simulink model "simulation_model_dynamic"  (R2024b)
settings: Solver=VariableStepAuto  StartTime=0.0  StopTime=100  MaxStep=1/60  RelTol=1e-3  EnableMultiTasking=on
values from neighbouring files (symbols this model uses):
  c_f = c_f*Cb    [fun00_GFL_pu_2_normial.m]    (also in fun00_GFM_pu_2_normial.m)
  fb = 60    [case_data.m]    (also in sim_m_case1.m; sim_m_case1_bench.m; sim_m_case2.m; sim_m_case2_bench.m)
  ki_i = ki_i_pu*Vb_p_ph/Ib_p_ph    [fun00_GFL_pu_2_normial.m]    (also in fun00_GFM_pu_2_normial.m)
  ki_p = ki_p_pu/Sb*Ib_p_ph    [fun00_GFL_pu_2_normial.m]
  ki_pll = ki_pll/Vb_p_ph    [fun00_GFL_pu_2_normial.m]
  ki_q = ki_q_pu/Sb*Ib_p_ph    [fun00_GFL_pu_2_normial.m]
  kp_i = kp_i_pu*Vb_p_ph/Ib_p_ph    [fun00_GFL_pu_2_normial.m]    (also in fun00_GFM_pu_2_normial.m)
  kp_p = kp_p_pu/Sb*Ib_p_ph    [fun00_GFL_pu_2_normial.m]
  kp_pll = kp_pll/Vb_p_ph    [fun00_GFL_pu_2_normial.m]
  kp_q = kp_q_pu/Sb*Ib_p_ph    [fun00_GFL_pu_2_normial.m]
  l_f = l_f*Lb    [fun00_GFL_pu_2_normial.m]    (also in fun00_GFM_pu_2_normial.m)
  line = mpc.line    [sim_m_case1.m]    (also in sim_m_case1_bench.m; sim_m_case2.m = mpc.line*1.1; sim_m_case2_bench.m = mpc.line*1.1; sim_m_case2_sparse.m = mpc.line*1.1)
  pset = p_set_pu*Sb    [fun00_GFL_pu_2_normial.m]
  qset = q_set_pu*Sb    [fun00_GFL_pu_2_normial.m]
  r_f = r_f*Zb    [fun00_GFL_pu_2_normial.m]    (also in fun00_GFM_pu_2_normial.m)
  Sb = 100*10^6    (= 100000000)    [sim_m_case1.m]    (also in sim_m_case1_bench.m; sim_m_case2.m; sim_m_case2_bench.m; sim_m_case2_sparse.m)
  t_gfl = 35    [sim_m_case1.m]    (also in sim_m_case1_bench.m = 30; sim_m_case2.m; sim_m_case2_bench.m = 30; sim_m_case2_sparse.m)
  t_gfm = 30    [sim_m_case1.m]    (also in sim_m_case1_bench.m; sim_m_case2.m; sim_m_case2_bench.m; sim_m_case2_sparse.m)
  trans_l = mpc.trans_l    [sim_m_case1.m]    (also in sim_m_case1_bench.m; sim_m_case2.m; sim_m_case2_bench.m; sim_m_case2_sparse.m)
  Vb_gfm = 20*10^3    (= 20000)    [sim_m_case1.m]    (also in sim_m_case1_bench.m; sim_m_case2.m; sim_m_case2_bench.m; sim_m_case2_sparse.m)
  Vb_h = 230*10^3    (= 230000)    [sim_m_case1.m]    (also in sim_m_case1_bench.m; sim_m_case2.m; sim_m_case2_bench.m; sim_m_case2_sparse.m)
  Vdc = 3*Vb_p_ph    [fun00_GFL_pu_2_normial.m]    (also in fun00_GFM_pu_2_normial.m)
  wb = 2*pi*fb    (= 376.991118431)    [case_data.m]    (also in sim_m_case1.m; sim_m_case1_bench.m; sim_m_case2.m; sim_m_case2_bench.m)
undefined symbols (not defined in the file or in its folder): c_f_gfm, d_gfl, D_p_gfm, D_p_gfm_s, D_q_gfm, DiscIntNeverNeededParam, Init, Init_GFL, J_gfm, ki_i_gfm, ki_pll_s, ki_vc_gfm, kp_i_gfm, kp_pll_s, kp_vc_gfm, l_f_gfm, P_set_gfm, Q_set_gfm, r_f_gfm, Vb, Vdc_gfm, VSM
libraries: spsThreePhaseVIMeasurementLib x52, spsabctodq0Lib x48, slpidlib x42, spsThreePhaseSeriesRLCBranchLib x36, spsFirstOrderFilterLib x16, spsThreePhaseTransformerTwoWindingsLib x9, spsGroundLib x9, spsPowerPositiveSequenceLib x9, spsdq0toabcLib x9, spsUniversalBridgeLib x9, spsDCVoltageSourceLib x9, spsThreePhaseSourceLib x5
(part 1 of 8)
settings Model: SimulationMode=accelerator  Creator=MathWorks  LastModifiedBy=victo
settings SolverCC: AlgebraicLoopSolver=TrustRegion
settings DataIOCC: SaveFormat=Array  SignalLoggingSaveFormat=ModelDataLogs  SaveOutput=off  SaveTime=off  ReturnWorkspaceOutputs=off  TimeSaveName=t  SignalLoggingName=sigsOut
settings OptimizationCC: BlockReduction=off  BooleanDataType=off  ExpressionDepthLimit=2147483647  InitFltsAndDblsToZero=on  LifeSpan=inf
settings DebuggingCC: UnderspecifiedInitializationDetection=Classic  MergeDetectMultiDrivingBlocksExec=none  SignalResolutionControl=TryResolveAllWithWarning  MultiTaskDSMMsg=warning  MultiTaskCondExecSysMsg=none  FcnCallInpInsideContextMsg=warning  StateNameClashWarn=warning  SFUnexpectedBacktrackingDiag=warning  SFNoUnconditionalDefaultTransitionDiag=warning  SFExecutionAtInitializationDiag=none  ArithmeticOperatorsInVariantConditions=warning
settings HardwareCC: ProdBitPerPointer=32  ProdBitPerSizeT=32  ProdBitPerPtrDiffT=32  ProdLargestAtomicFloat=None  ProdIntDivRoundTo=Undefined  ProdEndianess=Unspecified  ProdWordSize=32  ProdHWDeviceType=32-bit Generic  TargetBitPerPointer=64  TargetBitPerSizeT=64  TargetBitPerPtrDiffT=64  TargetLongLongMode=on  TargetIntDivRoundTo=Zero  TargetEndianess=LittleEndian  TargetWordSize=64  TargetHWDeviceType=MATLAB Host  ProdEqTarget=off
settings ModelReferenceCC: EnableRefExpFcnMdlSchedulingChecks=on  PropagateSignalLabelsOutOfModel=off
settings SFSimCC: SimUseLocalCustomCode=off  CustomCodeUndefinedFunction=UseInterfaceOnly
settings RTWCC: RTWUseLocalCustomCode=off  GPUComputeCapability=3.5
settings CodeAppCC: StateflowObjectComments=on
settings GRTTargetCC: TargetLangStandard=C89/C90 (ANSI)  CombineOutputUpdateFcns=off  GRTInterface=on
settings ConfigComp: CovMetricSettings=dw  CovSaveCumulativeToWorkspaceVar=on  CovSaveSingleToWorkspaceVar=on  CovExternalEMLEnable=off  CovSFcnEnable=off
settings SimscapeCC: SimscapeNormalizeSystem=off

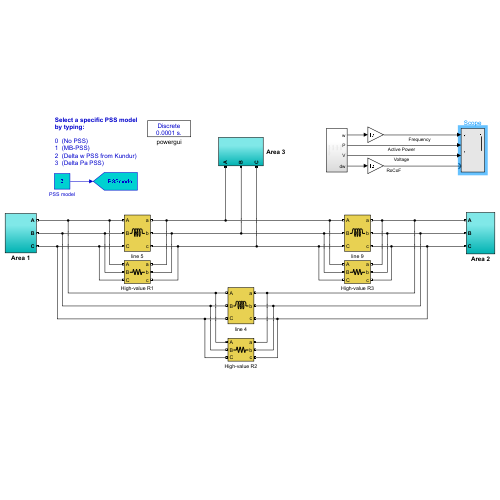
[thumbnail: Simulink's stored preview of the top-level diagram]
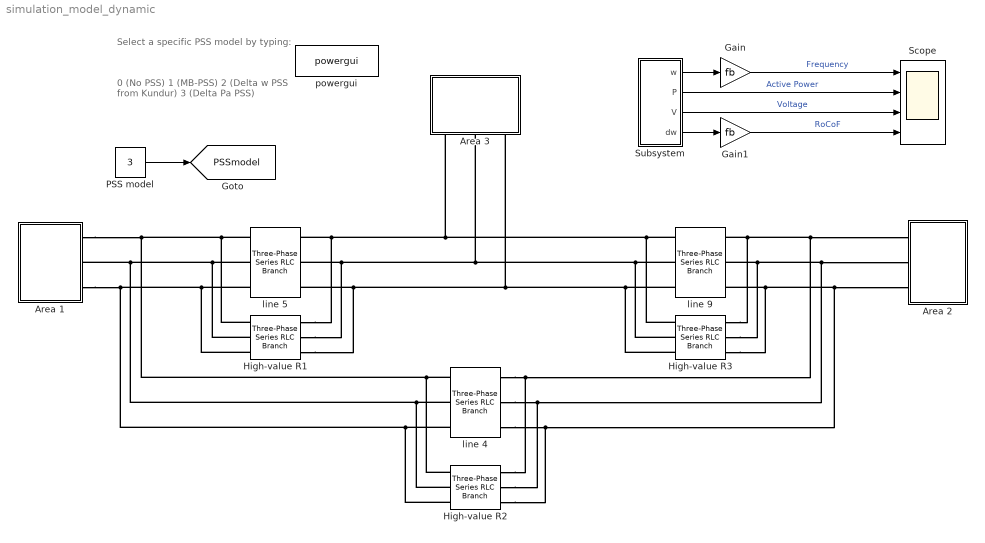
== system simulation_model_dynamic ==
  note: Select a specific PSS model
      | by typing:
  note: 0  (No PSS)
      | 1  (MB-PSS)
      | 2  (Delta w PSS from Kundur)
      | 3  (Delta Pa PSS)
  Area 1 : Subsystem
  Area 2 : Subsystem
  Area 3 : Subsystem
  Gain : Gain  Gain=fb
  Gain1 : Gain  Gain=fb
  High-value R1 : spsThreePhaseSeriesRLCBranchLib/Three-Phase Series RLC Branch  LConnTagsString=A|B|C  RConnTagsString=A|B|C  BranchType=R  Resistance=1e6  Inductance=line(3,4)  Capacitance=1e-6  Measurements=None
  High-value R2 : spsThreePhaseSeriesRLCBranchLib/Three-Phase Series RLC Branch  LConnTagsString=A|B|C  RConnTagsString=A|B|C  BranchType=R  Resistance=1e6  Inductance=line(3,4)  Capacitance=1e-6  Measurements=None
  High-value R3 : spsThreePhaseSeriesRLCBranchLib/Three-Phase Series RLC Branch  LConnTagsString=A|B|C  RConnTagsString=A|B|C  BranchType=R  Resistance=1e6  Inductance=line(3,4)  Capacitance=1e-6  Measurements=None
  PSS model : Constant  Value=3
  Scope : Scope  NumInputPorts=4
  Subsystem : Subsystem
  line 4 : spsThreePhaseSeriesRLCBranchLib/Three-Phase Series RLC Branch  LConnTagsString=A|B|C  RConnTagsString=A|B|C  BranchType=L  Resistance=line(14,3)  Inductance=line(4,4)  Capacitance=1e-6  Measurements=None
  line 5 : spsThreePhaseSeriesRLCBranchLib/Three-Phase Series RLC Branch  LConnTagsString=A|B|C  RConnTagsString=A|B|C  BranchType=L  Resistance=1e-4  Inductance=line(5,4)  Capacitance=1e-6  Measurements=None
  line 9 : spsThreePhaseSeriesRLCBranchLib/Three-Phase Series RLC Branch  LConnTagsString=A|B|C  RConnTagsString=A|B|C  BranchType=L  Resistance=line(14,3)  Inductance=line(9,4)  Capacitance=1e-6  Measurements=None
  powergui : sps_lib/powergui  Priority=2  SimulationMode=Discrete  SampleTime=1e-4  frequency=60  Iterations=1000  frequencyindice=0  Pbase=100e6  ErrMax=0.001  UnitsV=kV  UnitsW=MW  buscounter=0  FunctionMessages=off  echomessages=off  EnableUseOfTLC=off  CurrentSourceSwitches=off  DisableSnubberDevices=off  DisableRonSwitches=off  DisableVfSwitches=off  DisplayEquations=off  AutomaticDiscreteSolvers=off  SolverType=Tustin  Interpol=off  ExternalGateDelay=off  methode=off  Ts=0  x0status=steady  SPID=off  SwTol=0  HookPort=off  NonlinearTolerance=1e-4  nMaxIteration=100  ContinueOnMaxIteration=off  RestoreLinks=warning  ResistiveCurrentMeasurement=off  Frange=logspace(0,3,50)  Ylog=off  Xlog=off  ShowGrid=off  save=off  variable=ZData  structure=0  ZoomFFT=on  StartTime=0.0  cycles=1  DisplayStyle=1  fundamental=60  FreqAxis=off  MaxFrequency=1000  frequencyindicesteady=1  RmsSteady=2  display=off
  tag scope: PSSmodel=global
  wires:
  PSS model/1 -> [PSSmodel]
  Subsystem/2(P) -> Scope/2  "Active Power"
  Gain/1 -> Scope/1  "Frequency"
  Subsystem/3(V) -> Scope/3  "Voltage"
  Subsystem/1(w) -> Gain/1
  Subsystem/4(dw) -> Gain1/1
  Gain1/1 -> Scope/4  "RoCoF"
  connections:
  line 5/LConn2 -- High-value R1/LConn2 -- High-value R2/LConn2 -- line 4/LConn2 -- Area 1/RConn2
  line 5/LConn1 -- High-value R1/LConn1 -- High-value R2/LConn1 -- line 4/LConn1 -- Area 1/RConn1
  line 5/LConn3 -- High-value R1/LConn3 -- High-value R2/LConn3 -- line 4/LConn3 -- Area 1/RConn3
  line 4/RConn2 -- High-value R2/RConn2 -- Area 2/LConn2 -- High-value R3/RConn2 -- line 9/RConn2
  line 4/RConn1 -- High-value R2/RConn1 -- Area 2/LConn1 -- High-value R3/RConn1 -- line 9/RConn1
  line 4/RConn3 -- High-value R2/RConn3 -- Area 2/LConn3 -- High-value R3/RConn3 -- line 9/RConn3
  line 9/LConn2 -- High-value R3/LConn2 -- Area 3/LConn2 -- High-value R1/RConn2 -- line 5/RConn2
  line 9/LConn1 -- High-value R3/LConn1 -- Area 3/LConn1 -- High-value R1/RConn1 -- line 5/RConn1
  line 9/LConn3 -- High-value R3/LConn3 -- Area 3/LConn3 -- High-value R1/RConn3 -- line 5/RConn3

== system simulation_model_dynamic/Area 1 ==
  note: Area 1
  1 : spsThreePhaseVIMeasurementLib/Three-Phase V-I Measurement  VoltageMeasurement=phase-to-ground  SetLabelV=on  LabelV=Vabc_1  Vpu=off  VpuLL=off  CurrentMeasurement=no  SetLabelI=off  LabelI=Iabc  Ipu=off  Pbase=100e6  Vbase=500e3  OutputType=Complex  PhasorSimulation=off  PSBequivalent=0
  100MVA 20 kV-230 kV1 : spsThreePhaseTransformerTwoWindingsLib/Three-Phase Transformer (Two Windings)  Winding1Connection=Yg  Winding2Connection=Yg  CoreType=Three single-phase transformers  SetSaturation=off  Hysteresis=off  DataFile='hysteresis'  SetInitialFlux=off  Measurements=None  UNITS=pu  NominalPower="[ Sb   fb ]"  Winding1="[ 20e3  1e-6   0  ]"  Winding2="[ 230e3  1e-6   trans_l ]"  Rm=500  Lm=500  L0=0.5  Saturation="[ 0,0  ;  0.005,1.2  ;  1.0,1.4 ]"  InitialFluxes=[ 0.8 , -0.8 , 0.7 ]  BreakLoop=off  DiscreteSolver=Trapezoidal iterative  DataType=off  TransfoNumber=0
  100MVA 20 kV-230 kV2 : spsThreePhaseTransformerTwoWindingsLib/Three-Phase Transformer (Two Windings)  Winding1Connection=Yg  Winding2Connection=Yg  CoreType=Three single-phase transformers  SetSaturation=off  Hysteresis=off  DataFile='hysteresis'  SetInitialFlux=off  Measurements=None  UNITS=pu  NominalPower="[ Sb   fb ]"  Winding1="[ 20e3  1e-6   0  ]"  Winding2="[ 230e3  1e-6   trans_l ]"  Rm=500  Lm=500  L0=0.5  Saturation="[ 0,0  ;  0.005,1.2  ;  1.0,1.4 ]"  InitialFluxes=[ 0.8 , -0.8 , 0.7 ]  BreakLoop=off  DiscreteSolver=Trapezoidal iterative  DataType=off  TransfoNumber=0
  100MVA 20 kV-230 kV3 : spsThreePhaseTransformerTwoWindingsLib/Three-Phase Transformer (Two Windings)  Winding1Connection=Yg  Winding2Connection=Yg  CoreType=Three single-phase transformers  SetSaturation=off  Hysteresis=off  DataFile='hysteresis'  SetInitialFlux=off  Measurements=None  UNITS=pu  NominalPower="[Sb   fb ]"  Winding1="[ 20e3  1e-6   0  ]"  Winding2="[ 230e3  1e-6   trans_l ]"  Rm=500  Lm=500  L0=0.5  Saturation="[ 0,0  ;  0.005,1.2  ;  1.0,1.4 ]"  InitialFluxes=[ 0.8 , -0.8 , 0.7 ]  BreakLoop=off  DiscreteSolver=Trapezoidal iterative  DataType=off  TransfoNumber=0
  13 : spsThreePhaseVIMeasurementLib/Three-Phase V-I Measurement  VoltageMeasurement=phase-to-ground  SetLabelV=on  LabelV=Vabc_13  Vpu=off  VpuLL=off  CurrentMeasurement=no  SetLabelI=off  LabelI=Iabc  Ipu=off  Pbase=100e6  Vbase=500e3  OutputType=Complex  PhasorSimulation=off  PSBequivalent=0
  14 : spsThreePhaseVIMeasurementLib/Three-Phase V-I Measurement  VoltageMeasurement=phase-to-ground  SetLabelV=on  LabelV=Vabc_14  Vpu=off  VpuLL=off  CurrentMeasurement=no  SetLabelI=off  LabelI=Iabc  Ipu=off  Pbase=100e6  Vbase=500e3  OutputType=Complex  PhasorSimulation=off  PSBequivalent=0
  2 : spsThreePhaseVIMeasurementLib/Three-Phase V-I Measurement  VoltageMeasurement=phase-to-ground  SetLabelV=on  LabelV=Vabc_2  Vpu=off  VpuLL=off  CurrentMeasurement=no  SetLabelI=off  LabelI=Iabc  Ipu=off  Pbase=100e6  Vbase=500e3  OutputType=Complex  PhasorSimulation=off  PSBequivalent=0
  3 : spsThreePhaseVIMeasurementLib/Three-Phase V-I Measurement  VoltageMeasurement=phase-to-ground  SetLabelV=on  LabelV=Vabc_3  Vpu=off  VpuLL=off  CurrentMeasurement=no  SetLabelI=off  LabelI=Iabc  Ipu=off  Pbase=100e6  Vbase=500e3  OutputType=Complex  PhasorSimulation=off  PSBequivalent=0
  4 : spsThreePhaseVIMeasurementLib/Three-Phase V-I Measurement  VoltageMeasurement=phase-to-ground  SetLabelV=on  LabelV=Vabc_4  Vpu=off  VpuLL=off  CurrentMeasurement=no  SetLabelI=off  LabelI=Iabc  Ipu=off  Pbase=100e6  Vbase=500e3  OutputType=Complex  PhasorSimulation=off  PSBequivalent=0
  Bus Selector : BusSelector  OutputSignals="Mechanical.Rotor speed  wm  (pu),Output active power   Peo (pu),Output reactive power  Qeo (pu)"
  High-value R : spsThreePhaseSeriesRLCBranchLib/Three-Phase Series RLC Branch  LConnTagsString=A|B|C  RConnTagsString=A|B|C  BranchType=R  Resistance=1e6  Inductance=line(3,4)  Capacitance=1e-6  Measurements=None
  High-value R1 : spsThreePhaseSeriesRLCBranchLib/Three-Phase Series RLC Branch  LConnTagsString=A|B|C  RConnTagsString=A|B|C  BranchType=R  Resistance=1e6  Inductance=line(3,4)  Capacitance=1e-6  Measurements=None
  INVERTER 1 : Subsystem
  INVERTER 2 : Subsystem
  INVERTER 3 : Subsystem
  M1 100 MVA : spsSynchronousMachinepuStandardLib/Synchronous Machine pu Standard  PresetModel=No  MechanicalLoad=Mechanical power Pm  ShowDetailedParameters=on  RotorType=Round  Units=per unit standard parameters  MeasurementBus=off  NominalParameters="[100e6  20000   60 ]"  Reactances1=[1.8 .3 .25 1.7 .55 .25 .2]  Reactances2=[ 1.305, 0.296, 0.252, 0.474, 0.243, 0.18 ]  dAxisTimeConstants=Open-circuit  qAxisTimeConstants=Open-circuit  TimeConstants1=[]  TimeConstants2=[8 .03 .4 .05]  TimeConstants3=[]  TimeConstants4=[]  TimeConstants5=[ 1.01, 0.053, 0.1 ]  TimeConstants6=[]  TimeConstants7=[]  TimeConstants8=[]  StatorResistance=0.025  Mechanical=[1 0 4]  PolePairs=4  InitialConditions=[0 0 0 0 0 0 0 0 1.43051]  SetSaturation=off  Saturation=[0.6404,0.7127,0.8441,0.9214,0.9956,1.082,1.19,1.316,1.457;0.7,0.7698,0.8872,0.9466,0.9969,1.046,1.1,1.151,1.201]  LoadFlowParameters=[1 700000000 0 0 0]  TsPowergui=0  TsBlock=-1  IterativeModel=Trapezoidal non iterative  IterativeDiscreteModel=Trapezoidal non iterative  BusType=PV  Pref=50e6  Qref=0  Qmin=-Inf  Qmax=Inf  PLF=0  QLF=0
  M1: Turbine & Regulators : Subsystem
  Pref1 : Constant  Value=0.5
  Terminator : Terminator
  Terminator1 : Terminator
  Three-Phase Dynamic Load : spsThreePhaseDynamicLoadLib/Three-Phase Dynamic Load  NominalVoltage=[ Vb_h fb ]  ActiveReactivePowers=[400e6 0]  PositiveSequence=[1 0]  ExternalControl=off  NpNq=[0.7473 0.7268]  TimeConstants="[0  0.011  0  0.0366]"  MinimumVoltage=0.5  Tfilter=1e-4  LoadFlowParameters=[4,0,0,0,0]
      settings: LibrarySourceBlock=|
      | sps_lib/Passives/Three-Phase
      | Dynamic Load
  Three-Phase Dynamic Load1 : spsThreePhaseDynamicLoadLib/Three-Phase Dynamic Load  NominalVoltage=[ Vb_h fb ]  ActiveReactivePowers=[581e6 -100e6]  PositiveSequence=[0.994 -11.8]  ExternalControl=off  NpNq=[0.7473 0.7268]  TimeConstants="[0  0.011  0  0.0366]"  MinimumVoltage=0.5  Tfilter=1e-4  LoadFlowParameters=[4,0,0,0,0]
      settings: LibrarySourceBlock=|
      | sps_lib/Passives/Three-Phase
      | Dynamic Load
  Vref11 : Constant
  line 1 : spsThreePhaseSeriesRLCBranchLib/Three-Phase Series RLC Branch  LConnTagsString=A|B|C  RConnTagsString=A|B|C  BranchType=L  Resistance=1e-4  Inductance=line(1,4)  Capacitance=1e-6  Measurements=None
  line 3 : spsThreePhaseSeriesRLCBranchLib/Three-Phase Series RLC Branch  LConnTagsString=A|B|C  RConnTagsString=A|B|C  BranchType=L  Resistance=1e-4  Inductance=line(3,4)  Capacitance=1e-6  Measurements=None
  " A" : PMIOPort  Side=Right
  " B" : PMIOPort  Port=2  Side=Right
  " C" : PMIOPort  Port=3  Side=Right
  tag scope: P_sm1=global, Q_sm1=global, w_sm1=global
  wires:
  Pref1/1 -> M1: Turbine & Regulators/2(Pref)
  [PSSmodel] -> M1: Turbine & Regulators/4(PSS)
  M1: Turbine & Regulators/1(Pm) -> M1 100 MVA/1
  M1: Turbine & Regulators/2(Vf) -> M1 100 MVA/2
  Vref11/1 -> M1: Turbine & Regulators/3(Vref)
  M1 100 MVA/1 -> M1: Turbine & Regulators/1(m), Bus Selector/1
  Bus Selector/1 -> [w_sm1]  "<Rotor speed  wm  (pu)>"
  Bus Selector/2 -> [P_sm1]  "<Output active power   Peo (pu)>"
  Bus Selector/3 -> [Q_sm1]  "<Output reactive power  Qeo (pu)>"
  Three-Phase Dynamic Load/1 -> Terminator/1
  Three-Phase Dynamic Load1/1 -> Terminator1/1
  connections:
  2/LConn1 -- INVERTER 2/LConn1
  2/LConn3 -- INVERTER 2/LConn3
  100MVA 20 kV-230 kV3/RConn1 -- Three-Phase Dynamic Load1/LConn1 -- 4/LConn1 -- High-value R/RConn1 -- line 3/RConn1
  Three-Phase Dynamic Load1/LConn2 -- 4/LConn2 -- 100MVA 20 kV-230 kV3/RConn2 -- High-value R/RConn2 -- line 3/RConn2
  4/LConn3 -- Three-Phase Dynamic Load1/LConn3 -- 100MVA 20 kV-230 kV3/RConn3 -- High-value R/RConn3 -- line 3/RConn3
  INVERTER 1/LConn1 -- 13/LConn1
  INVERTER 1/LConn2 -- 13/LConn2
  INVERTER 1/LConn3 -- 13/LConn3
  line 3/LConn2 -- High-value R/LConn2 -- Three-Phase Dynamic Load/LConn2 -- 3/RConn2
  line 3/LConn1 -- High-value R/LConn1 -- Three-Phase Dynamic Load/LConn1 -- 3/RConn1
  3/LConn3 -- 100MVA 20 kV-230 kV2/RConn3 -- High-value R1/RConn3 -- line 1/RConn3
  2/LConn2 -- INVERTER 2/LConn2
  1/LConn1 -- 100MVA 20 kV-230 kV1/RConn1
  1/LConn2 -- 100MVA 20 kV-230 kV1/RConn2
  1/LConn3 -- 100MVA 20 kV-230 kV1/RConn3
  3/LConn1 -- 100MVA 20 kV-230 kV2/RConn1 -- High-value R1/RConn1 -- line 1/RConn1
  line 3/LConn3 -- High-value R/LConn3 -- Three-Phase Dynamic Load/LConn3 -- 3/RConn3
  3/LConn2 -- 100MVA 20 kV-230 kV2/RConn2 -- High-value R1/RConn2 -- line 1/RConn2
  100MVA 20 kV-230 kV1/LConn3 -- M1 100 MVA/RConn3 -- 13/RConn3
  100MVA 20 kV-230 kV1/LConn2 -- M1 100 MVA/RConn2 -- 13/RConn2
  100MVA 20 kV-230 kV1/LConn1 -- M1 100 MVA/RConn1 -- 13/RConn1
  100MVA 20 kV-230 kV2/LConn2 -- 2/RConn2
  100MVA 20 kV-230 kV2/LConn1 -- 2/RConn1
  100MVA 20 kV-230 kV2/LConn3 -- 2/RConn3
  4/RConn1 -- " A"/RConn1
  " B"/RConn1 -- 4/RConn2
  " C"/RConn1 -- 4/RConn3
  1/RConn1 -- High-value R1/LConn1 -- line 1/LConn1
  1/RConn2 -- High-value R1/LConn2 -- line 1/LConn2
  1/RConn3 -- High-value R1/LConn3 -- line 1/LConn3
  14/LConn1 -- INVERTER 3/LConn1
  14/LConn2 -- INVERTER 3/LConn2
  14/LConn3 -- INVERTER 3/LConn3
  14/RConn1 -- 100MVA 20 kV-230 kV3/LConn1
  100MVA 20 kV-230 kV3/LConn2 -- 14/RConn2
  14/RConn3 -- 100MVA 20 kV-230 kV3/LConn3

== system simulation_model_dynamic/Area 2 ==
  note: Area 2
  15 : spsThreePhaseVIMeasurementLib/Three-Phase V-I Measurement  VoltageMeasurement=phase-to-ground  SetLabelV=on  LabelV=Vabc_15  Vpu=off  VpuLL=off  CurrentMeasurement=no  SetLabelI=off  LabelI=Iabc  Ipu=off  Pbase=100e6  Vbase=500e3  OutputType=Complex  PhasorSimulation=off  PSBequivalent=0
  5 : spsThreePhaseVIMeasurementLib/Three-Phase V-I Measurement  VoltageMeasurement=phase-to-ground  SetLabelV=on  LabelV=Vabc_5  Vpu=off  VpuLL=off  CurrentMeasurement=no  SetLabelI=off  LabelI=Iabc  Ipu=off  Pbase=100e6  Vbase=500e3  OutputType=Complex  PhasorSimulation=off  PSBequivalent=0
  6 : spsThreePhaseVIMeasurementLib/Three-Phase V-I Measurement  VoltageMeasurement=phase-to-ground  SetLabelV=on  LabelV=Vabc_6  Vpu=off  VpuLL=off  CurrentMeasurement=no  SetLabelI=off  LabelI=Iabc  Ipu=off  Pbase=100e6  Vbase=500e3  OutputType=Complex  PhasorSimulation=off  PSBequivalent=0
  7 : spsThreePhaseVIMeasurementLib/Three-Phase V-I Measurement  VoltageMeasurement=phase-to-ground  SetLabelV=on  LabelV=Vabc_7  Vpu=off  VpuLL=off  CurrentMeasurement=no  SetLabelI=off  LabelI=Iabc  Ipu=off  Pbase=100e6  Vbase=500e3  OutputType=Complex  PhasorSimulation=off  PSBequivalent=0
  8 : spsThreePhaseVIMeasurementLib/Three-Phase V-I Measurement  VoltageMeasurement=phase-to-ground  SetLabelV=on  LabelV=Vabc_8  Vpu=off  VpuLL=off  CurrentMeasurement=no  SetLabelI=off  LabelI=Iabc  Ipu=off  Pbase=100e6  Vbase=500e3  OutputType=Complex  PhasorSimulation=off  PSBequivalent=0
  Bus Selector : BusSelector  OutputSignals="Mechanical.Rotor speed  wm  (pu),Output active power   Peo (pu),Output reactive power  Qeo (pu)"
  High-value R1 : spsThreePhaseSeriesRLCBranchLib/Three-Phase Series RLC Branch  LConnTagsString=A|B|C  RConnTagsString=A|B|C  BranchType=R  Resistance=1e6  Inductance=line(3,4)  Capacitance=1e-6  Measurements=None
  High-value R3 : spsThreePhaseSeriesRLCBranchLib/Three-Phase Series RLC Branch  LConnTagsString=A|B|C  RConnTagsString=A|B|C  BranchType=R  Resistance=1e6  Inductance=line(3,4)  Capacitance=1e-6  Measurements=None
  INVERTER 4 : Subsystem
  INVERTER 5 : Subsystem
  INVERTER 6 : Subsystem
  M6 900 MVA : spsSynchronousMachinepuStandardLib/Synchronous Machine pu Standard  PresetModel=No  MechanicalLoad=Mechanical power Pm  ShowDetailedParameters=on  RotorType=Round  Units=per unit standard parameters  MeasurementBus=off  NominalParameters="[100E6  20000   60 ]"  Reactances1=[1.8 .3 .25 1.7 .55 .25 .2]  Reactances2=[ 1.305, 0.296, 0.252, 0.474, 0.243, 0.18 ]  dAxisTimeConstants=Open-circuit  qAxisTimeConstants=Open-circuit  TimeConstants1=[]  TimeConstants2=[8 .03 .4 .05]  TimeConstants3=[]  TimeConstants4=[]  TimeConstants5=[ 1.01, 0.053, 0.1 ]  TimeConstants6=[]  TimeConstants7=[]  TimeConstants8=[]  StatorResistance=0.025  Mechanical=[1 0 4]  PolePairs=4  InitialConditions=[0 0 0 0 0 0 0 0 1.39666]  SetSaturation=off  Saturation=[0.6404,0.7127,0.8441,0.9214,0.9956,1.082,1.19,1.316,1.457;0.7,0.7698,0.8872,0.9466,0.9969,1.046,1.1,1.151,1.201]  LoadFlowParameters=[1 700000000 0 0 0]  TsPowergui=0  TsBlock=-1  IterativeModel=Trapezoidal non iterative  IterativeDiscreteModel=Trapezoidal non iterative  BusType=PV  Pref=50e6  Qref=0  Qmin=-Inf  Qmax=Inf  PLF=0  QLF=0
  M6: Turbine & Regulators : Subsystem
  Pref6 : Constant  Value=0.5
  T1: 100MVA 20 kV-230 kV : spsThreePhaseTransformerTwoWindingsLib/Three-Phase Transformer (Two Windings)  Winding1Connection=Yg  Winding2Connection=Yg  CoreType=Three single-phase transformers  SetSaturation=off  Hysteresis=off  DataFile='hysteresis'  SetInitialFlux=off  Measurements=None  UNITS=pu  NominalPower="[Sb   fb ]"  Winding1="[ 20e3  1e-6   0  ]"  Winding2="[ 230e3  1e-6   trans_l ]"  Rm=500  Lm=500  L0=0.5  Saturation="[ 0,0  ;  0.005,1.2  ;  1.0,1.4 ]"  InitialFluxes=[ 0.8 , -0.8 , 0.7 ]  BreakLoop=off  DiscreteSolver=Trapezoidal iterative  DataType=off  TransfoNumber=0
  T1: 900MVA 20 kV-230 kV1 : spsThreePhaseTransformerTwoWindingsLib/Three-Phase Transformer (Two Windings)  Winding1Connection=Yg  Winding2Connection=Yg  CoreType=Three single-phase transformers  SetSaturation=off  Hysteresis=off  DataFile='hysteresis'  SetInitialFlux=off  Measurements=None  UNITS=pu  NominalPower="[ 100e6   60 ]"  Winding1="[ 20e3  1e-6   0  ]"  Winding2="[ 230e3  1e-6   trans_l ]"  Rm=500  Lm=500  L0=0.5  Saturation="[ 0,0  ;  0.005,1.2  ;  1.0,1.4 ]"  InitialFluxes=[ 0.8 , -0.8 , 0.7 ]  BreakLoop=off  DiscreteSolver=Trapezoidal iterative  DataType=off  TransfoNumber=0
  T1: 900MVA 20 kV-230 kV2 : spsThreePhaseTransformerTwoWindingsLib/Three-Phase Transformer (Two Windings)  Winding1Connection=Yg  Winding2Connection=Yg  CoreType=Three single-phase transformers  SetSaturation=off  Hysteresis=off  DataFile='hysteresis'  SetInitialFlux=off  Measurements=None  UNITS=pu  NominalPower="[ 100e6   60 ]"  Winding1="[ 20e3  1e-6   0  ]"  Winding2="[ 230e3  1e-6   trans_l ]"  Rm=500  Lm=500  L0=0.5  Saturation="[ 0,0  ;  0.005,1.2  ;  1.0,1.4 ]"  InitialFluxes=[ 0.8 , -0.8 , 0.7 ]  BreakLoop=off  DiscreteSolver=Trapezoidal iterative  DataType=off  TransfoNumber=0
  Terminator : Terminator
  Terminator1 : Terminator
  Three-Phase Dynamic Load : spsThreePhaseDynamicLoadLib/Three-Phase Dynamic Load  NominalVoltage=[ Vb_h fb ]  ActiveReactivePowers=[490e6 0]  PositiveSequence=[0.994 -11.8]  ExternalControl=off  NpNq=[2 2]  TimeConstants="[0  0.011  0  0.0366]"  MinimumVoltage=0.5  Tfilter=1e-4  LoadFlowParameters=[4,0,0,0,0]
      settings: LibrarySourceBlock=|
      | sps_lib/Passives/Three-Phase
      | Dynamic Load
  Three-Phase Dynamic Load1 : spsThreePhaseDynamicLoadLib/Three-Phase Dynamic Load  NominalVoltage=[ Vb_h fb ]  ActiveReactivePowers=[1000e6 -250e6]  PositiveSequence=[0.994 -11.8]  ExternalControl=off  NpNq=[1.9 2.1]  TimeConstants="[0  0  0  0]"  MinimumVoltage=0.5  Tfilter=1e-4  LoadFlowParameters=[4,0,0,0,0]
      settings: LibrarySourceBlock=|
      | sps_lib/Passives/Three-Phase
      | Dynamic Load
  Vref6 : Constant
  line 6 : spsThreePhaseSeriesRLCBranchLib/Three-Phase Series RLC Branch  LConnTagsString=A|B|C  RConnTagsString=A|B|C  BranchType=L  Resistance=line(14,3)  Inductance=line(6,4)  Capacitance=1e-6  Measurements=None
  line 8 : spsThreePhaseSeriesRLCBranchLib/Three-Phase Series RLC Branch  LConnTagsString=A|B|C  RConnTagsString=A|B|C  BranchType=L  Resistance=line(14,3)  Inductance=line(8,4)  Capacitance=1e-6  Measurements=None
  A : PMIOPort  Side=Left
  B : PMIOPort  Port=2  Side=Left
  C : PMIOPort  Port=3  Side=Left
  tag scope: P_sm2=global, Q_sm2=global, w_sm2=global
  wires:
  [PSSmodel] -> M6: Turbine & Regulators/4(PSS)
  Pref6/1 -> M6: Turbine & Regulators/2(Pref)
  Vref6/1 -> M6: Turbine & Regulators/3(Vref)
  M6: Turbine & Regulators/1(Pm) -> M6 900 MVA/1
  M6: Turbine & Regulators/2(Vf) -> M6 900 MVA/2
  M6 900 MVA/1 -> Bus Selector/1, M6: Turbine & Regulators/1(m)
  Bus Selector/2 -> [P_sm2]  "<Output active power   Peo (pu)>"
  Bus Selector/1 -> [w_sm2]  "<Rotor speed  wm  (pu)>"
  Bus Selector/3 -> [Q_sm2]  "<Output reactive power  Qeo (pu)>"
  Three-Phase Dynamic Load/1 -> Terminator/1
  Three-Phase Dynamic Load1/1 -> Terminator1/1
  connections:
  5/LConn1 -- INVERTER 4/LConn1
  line 6/LConn3 -- High-value R3/LConn3 -- T1: 100MVA 20 kV-230 kV/RConn3
  6/LConn1 -- INVERTER 5/LConn1
  line 6/LConn2 -- High-value R3/LConn2 -- T1: 100MVA 20 kV-230 kV/RConn2
  line 6/LConn1 -- High-value R3/LConn1 -- T1: 100MVA 20 kV-230 kV/RConn1
  T1: 900MVA 20 kV-230 kV1/RConn2 -- Three-Phase Dynamic Load/LConn2 -- High-value R3/RConn2 -- line 6/RConn2 -- 7/LConn2
  T1: 900MVA 20 kV-230 kV1/RConn1 -- Three-Phase Dynamic Load/LConn1 -- High-value R3/RConn1 -- line 6/RConn1 -- 7/LConn1
  T1: 900MVA 20 kV-230 kV1/RConn3 -- Three-Phase Dynamic Load/LConn3 -- 7/LConn3 -- High-value R3/RConn3 -- line 6/RConn3
  8/LConn1 -- High-value R1/RConn1 -- line 8/RConn1 -- Three-Phase Dynamic Load1/LConn1 -- T1: 900MVA 20 kV-230 kV2/RConn1
  8/LConn2 -- High-value R1/RConn2 -- line 8/RConn2 -- Three-Phase Dynamic Load1/LConn2 -- T1: 900MVA 20 kV-230 kV2/RConn2
  T1: 900MVA 20 kV-230 kV2/RConn3 -- High-value R1/RConn3 -- line 8/RConn3 -- Three-Phase Dynamic Load1/LConn3 -- 8/LConn3
  5/LConn2 -- INVERTER 4/LConn2
  5/LConn3 -- INVERTER 4/LConn3
  6/LConn2 -- INVERTER 5/LConn2
  6/LConn3 -- INVERTER 5/LConn3
  15/LConn3 -- INVERTER 6/LConn3
  15/LConn2 -- INVERTER 6/LConn2
  15/LConn1 -- INVERTER 6/LConn1
  T1: 900MVA 20 kV-230 kV2/LConn1 -- 15/RConn1
  T1: 900MVA 20 kV-230 kV2/LConn3 -- 15/RConn3
  T1: 900MVA 20 kV-230 kV2/LConn2 -- 15/RConn2
  8/RConn1 -- A/RConn1
  8/RConn2 -- B/RConn1
  C/RConn1 -- 8/RConn3
  7/RConn1 -- High-value R1/LConn1 -- line 8/LConn1
  7/RConn2 -- High-value R1/LConn2 -- line 8/LConn2
  7/RConn3 -- High-value R1/LConn3 -- line 8/LConn3
  5/RConn1 -- T1: 100MVA 20 kV-230 kV/LConn1
  T1: 100MVA 20 kV-230 kV/LConn2 -- 5/RConn2
  5/RConn3 -- T1: 100MVA 20 kV-230 kV/LConn3
  6/RConn1 -- M6 900 MVA/RConn1 -- T1: 900MVA 20 kV-230 kV1/LConn1
  T1: 900MVA 20 kV-230 kV1/LConn2 -- M6 900 MVA/RConn2 -- 6/RConn2
  T1: 900MVA 20 kV-230 kV1/LConn3 -- M6 900 MVA/RConn3 -- 6/RConn3

== system simulation_model_dynamic/Area 3 ==
  note: Area 3
  10 : spsThreePhaseVIMeasurementLib/Three-Phase V-I Measurement  VoltageMeasurement=phase-to-ground  SetLabelV=on  LabelV=Vabc_10  Vpu=off  VpuLL=off  CurrentMeasurement=no  SetLabelI=off  LabelI=Iabc  Ipu=off  Pbase=100e6  Vbase=500e3  OutputType=Complex  PhasorSimulation=off  PSBequivalent=0
  11 : spsThreePhaseVIMeasurementLib/Three-Phase V-I Measurement  VoltageMeasurement=phase-to-ground  SetLabelV=on  LabelV=Vabc_11  Vpu=off  VpuLL=off  CurrentMeasurement=no  SetLabelI=off  LabelI=Iabc  Ipu=off  Pbase=100e6  Vbase=500e3  OutputType=Complex  PhasorSimulation=off  PSBequivalent=0
  12 : spsThreePhaseVIMeasurementLib/Three-Phase V-I Measurement  VoltageMeasurement=phase-to-ground  SetLabelV=on  LabelV=Vabc_12  Vpu=off  VpuLL=off  CurrentMeasurement=no  SetLabelI=off  LabelI=Iabc  Ipu=off  Pbase=100e6  Vbase=500e3  OutputType=Complex  PhasorSimulation=off  PSBequivalent=0
  1570MW : spsThreePhaseParallelRLCLoadLib/Three-Phase Parallel RLC Load  LConnTagsString=A|B|C  Configuration=Y (grounded)  NominalVoltage=(230000)*0.975891  Vabc=[1e3 1e3 1e3]  Vabcp=[1e3 1e3 1e3]  NominalFrequency=60  UnbalancedPower=off  ActivePower=1570e6  InductivePower=0  CapacitivePower=0  Pabc=[10e3 9e3 11e3]  QLabc=[100 90 110]  QCabc=[100 90 110]  Pabcp=[10e3 9e3 11e3]  QLabcp=[100 90 110]  QCabcp=[100 90 110]  Measurements=None  LoadType=constant PQ
  16 : spsThreePhaseVIMeasurementLib/Three-Phase V-I Measurement  VoltageMeasurement=phase-to-ground  SetLabelV=on  LabelV=Vabc_17  Vpu=off  VpuLL=off  CurrentMeasurement=no  SetLabelI=off  LabelI=Iabc  Ipu=off  Pbase=100e6  Vbase=500e3  OutputType=Complex  PhasorSimulation=off  PSBequivalent=0
  300MW : spsThreePhaseParallelRLCLoadLib/Three-Phase Parallel RLC Load  LConnTagsString=A|B|C  Configuration=Y (grounded)  NominalVoltage=230e3  Vabc=[1e3 1e3 1e3]  Vabcp=[1e3 1e3 1e3]  NominalFrequency=60  UnbalancedPower=off  ActivePower=300e6  InductivePower=0  CapacitivePower=0  Pabc=[10e3 9e3 11e3]  QLabc=[100 90 110]  QCabc=[100 90 110]  Pabcp=[10e3 9e3 11e3]  QLabcp=[100 90 110]  QCabcp=[100 90 110]  Measurements=None  LoadType=constant PQ
  9 : spsThreePhaseVIMeasurementLib/Three-Phase V-I Measurement  VoltageMeasurement=phase-to-ground  SetLabelV=on  LabelV=Vabc_9  Vpu=off  VpuLL=off  CurrentMeasurement=no  SetLabelI=off  LabelI=Iabc  Ipu=off  Pbase=100e6  Vbase=500e3  OutputType=Complex  PhasorSimulation=off  PSBequivalent=0
  900MVA 20 kV-230 kV3 : spsThreePhaseTransformerTwoWindingsLib/Three-Phase Transformer (Two Windings)  Winding1Connection=Yg  Winding2Connection=Yg  CoreType=Three single-phase transformers  SetSaturation=off  Hysteresis=off  DataFile='hysteresis'  SetInitialFlux=off  Measurements=None  UNITS=pu  NominalPower="[ 100e6   60 ]"  Winding1="[ 20e3  1e-6   0  ]"  Winding2="[ 230e3  1e-6   trans_l ]"  Rm=500  Lm=500  L0=0.5  Saturation="[ 0,0  ;  0.005,1.2  ;  1.0,1.4 ]"  InitialFluxes=[ 0.8 , -0.8 , 0.7 ]  BreakLoop=off  DiscreteSolver=Trapezoidal iterative  DataType=off  TransfoNumber=0
  High-value R1 : spsThreePhaseSeriesRLCBranchLib/Three-Phase Series RLC Branch  LConnTagsString=A|B|C  RConnTagsString=A|B|C  BranchType=R  Resistance=1e6  Inductance=line(3,4)  Capacitance=1e-6  Measurements=None
  High-value R2 : spsThreePhaseSeriesRLCBranchLib/Three-Phase Series RLC Branch  LConnTagsString=A|B|C  RConnTagsString=A|B|C  BranchType=R  Resistance=1e6  Inductance=line(3,4)  Capacitance=1e-6  Measurements=None
  INVERTER 7 : Subsystem
  INVERTER 8 : Subsystem
  INVERTER 9 : Subsystem
  T9: 900MVA 20 kV-230 kV1 : spsThreePhaseTransformerTwoWindingsLib/Three-Phase Transformer (Two Windings)  Winding1Connection=Yg  Winding2Connection=Yg  CoreType=Three single-phase transformers  SetSaturation=off  Hysteresis=off  DataFile='hysteresis'  SetInitialFlux=off  Measurements=None  UNITS=pu  NominalPower="[ 100e6   60 ]"  Winding1="[ 20e3  1e-6   0  ]"  Winding2="[ 230e3  1e-6   trans_l ]"  Rm=500  Lm=500  L0=0.5  Saturation="[ 0,0  ;  0.005,1.2  ;  1.0,1.4 ]"  InitialFluxes=[ 0.8 , -0.8 , 0.7 ]  BreakLoop=off  DiscreteSolver=Trapezoidal iterative  DataType=off  TransfoNumber=0
  T9: 900MVA 20 kV-230 kV2 : spsThreePhaseTransformerTwoWindingsLib/Three-Phase Transformer (Two Windings)  Winding1Connection=Yg  Winding2Connection=Yg  CoreType=Three single-phase transformers  SetSaturation=off  Hysteresis=off  DataFile='hysteresis'  SetInitialFlux=off  Measurements=None  UNITS=pu  NominalPower="[ 100e6   60 ]"  Winding1="[ 20e3  1e-6   0  ]"  Winding2="[ 230e3  1e-6   trans_l ]"  Rm=500  Lm=500  L0=0.5  Saturation="[ 0,0  ;  0.005,1.2  ;  1.0,1.4 ]"  InitialFluxes=[ 0.8 , -0.8 , 0.7 ]  BreakLoop=off  DiscreteSolver=Trapezoidal iterative  DataType=off  TransfoNumber=0
  Three-Phase Breaker : spsThreePhaseBreakerLib/Three-Phase Breaker  InitialState=open  SwitchA=on  SwitchB=on  SwitchC=on  SwitchTimes=40  External=off  BreakerResistance=0.01  SnubberResistance=1e6  SnubberCapacitance=inf  Measurements=None
  line 10 : spsThreePhaseSeriesRLCBranchLib/Three-Phase Series RLC Branch  LConnTagsString=A|B|C  RConnTagsString=A|B|C  BranchType=L  Resistance=line(14,3)  Inductance=line(10,4)  Capacitance=1e-6  Measurements=None
  line 12 : spsThreePhaseSeriesRLCBranchLib/Three-Phase Series RLC Branch  LConnTagsString=A|B|C  RConnTagsString=A|B|C  BranchType=L  Resistance=line(14,3)  Inductance=line(12,4)  Capacitance=1e-6  Measurements=None
  A : PMIOPort  Side=Left
  B : PMIOPort  Port=2  Side=Left
  C : PMIOPort  Port=3  Side=Left
  connections:
  9/LConn1 -- INVERTER 7/LConn1
  900MVA 20 kV-230 kV3/RConn3 -- High-value R1/LConn1 -- line 10/LConn3
  10/LConn1 -- INVERTER 8/LConn1
  900MVA 20 kV-230 kV3/RConn2 -- High-value R1/LConn2 -- line 10/LConn2
  900MVA 20 kV-230 kV3/RConn1 -- High-value R1/LConn3 -- line 10/LConn1
  Three-Phase Breaker/LConn2 -- High-value R2/LConn2 -- 11/RConn2 -- line 12/LConn2
  Three-Phase Breaker/LConn3 -- High-value R2/LConn3 -- 11/RConn3 -- line 12/LConn3
  line 12/RConn1 -- High-value R2/RConn1 -- 1570MW/LConn1 -- 12/LConn1
  B/RConn1 -- 12/RConn2 -- T9: 900MVA 20 kV-230 kV2/RConn2
  C/RConn1 -- 12/RConn3 -- T9: 900MVA 20 kV-230 kV2/RConn3
  9/LConn3 -- INVERTER 7/LConn3
  9/LConn2 -- INVERTER 7/LConn2
  10/LConn2 -- INVERTER 8/LConn2
  10/LConn3 -- INVERTER 8/LConn3
  T9: 900MVA 20 kV-230 kV1/LConn1 -- 10/RConn1
  T9: 900MVA 20 kV-230 kV1/LConn2 -- 10/RConn2
  T9: 900MVA 20 kV-230 kV1/LConn3 -- 10/RConn3
  Three-Phase Breaker/RConn1 -- 300MW/LConn1
  Three-Phase Breaker/RConn2 -- 300MW/LConn2
  Three-Phase Breaker/RConn3 -- 300MW/LConn3
  line 12/LConn1 -- High-value R2/LConn1 -- 11/RConn1 -- Three-Phase Breaker/LConn1
  16/LConn3 -- INVERTER 9/LConn3
  16/LConn2 -- INVERTER 9/LConn2
  16/LConn1 -- INVERTER 9/LConn1
  T9: 900MVA 20 kV-230 kV2/LConn1 -- 16/RConn1
  T9: 900MVA 20 kV-230 kV2/LConn3 -- 16/RConn3
  T9: 900MVA 20 kV-230 kV2/LConn2 -- 16/RConn2
  line 12/RConn3 -- 1570MW/LConn3 -- High-value R2/RConn3 -- 12/LConn3
  line 12/RConn2 -- 1570MW/LConn2 -- High-value R2/RConn2 -- 12/LConn2
  A/RConn1 -- 12/RConn1 -- T9: 900MVA 20 kV-230 kV2/RConn1
  T9: 900MVA 20 kV-230 kV1/RConn1 -- 11/LConn1 -- High-value R1/RConn3 -- line 10/RConn1
  line 10/RConn2 -- High-value R1/RConn2 -- 11/LConn2 -- T9: 900MVA 20 kV-230 kV1/RConn2
  line 10/RConn3 -- High-value R1/RConn1 -- 11/LConn3 -- T9: 900MVA 20 kV-230 kV1/RConn3
  9/RConn1 -- 900MVA 20 kV-230 kV3/LConn1
  900MVA 20 kV-230 kV3/LConn2 -- 9/RConn2
  9/RConn3 -- 900MVA 20 kV-230 kV3/LConn3

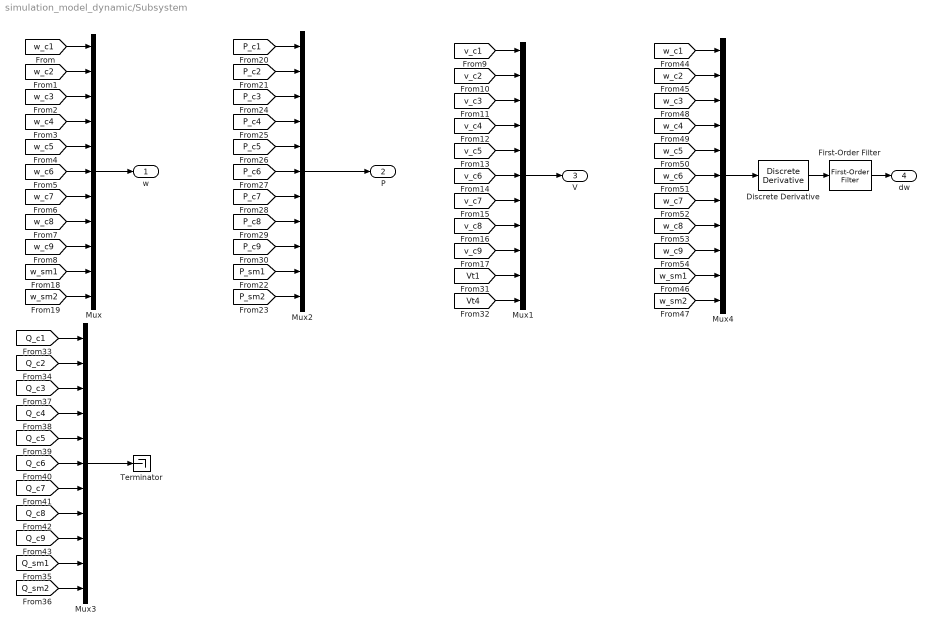
== system simulation_model_dynamic/Subsystem ==
  Discrete Derivative : simulink/Quick Insert/Discrete/Discrete Derivative  gainval=1.0  ICPrevScaledInput=0.0  OutMin=[]  OutMax=[]  OutDataType=fixdt(1, 16)  OutScaling=2^-10  DoSatur=off
  First-Order Filter : spsFirstOrderFilterLib/First-Order Filter  FilterType=Lowpass  Tc=0.1  Ts=0  Initialize=on  Vac_Init=[0, 0, 0]  Vdc_Init=0  PlotResponse=off  FreqRange="[0,  200,  1]"
  Mux{,1..4} (5 alike) : Mux  Inputs=11
  Terminator : Terminator
  w : Outport
  P : Outport  Port=2
  V : Outport  Port=3
  dw : Outport  Port=4
  wires:
  [P_sm2] -> Mux2/11
  [v_c8] -> Mux1/8
  [Q_c1] -> Mux3/1
  [Q_sm1] -> Mux3/10
  [Q_c7] -> Mux3/7
  [Q_c6] -> Mux3/6
  [w_c5] -> Mux/5
  [Q_c2] -> Mux3/2
  [Q_c5] -> Mux3/5
  [Q_c9] -> Mux3/9
  [v_c2] -> Mux1/2
  [P_c5] -> Mux2/5
  [Q_c8] -> Mux3/8
  [w_sm2] -> Mux/11
  [Q_sm2] -> Mux3/11
  [P_c4] -> Mux2/4
  Mux2/1 -> P/1
  [P_c7] -> Mux2/7
  [Q_c3] -> Mux3/3
  [Q_c4] -> Mux3/4
  [w_c7] -> Mux/7
  [w_c4] -> Mux/4
  [w_c2] -> Mux/2
  [v_c3] -> Mux1/3
  [v_c4] -> Mux1/4
  [w_c6] -> Mux/6
  [v_c7] -> Mux1/7
  [v_c9] -> Mux1/9
  [v_c5] -> Mux1/5
  [w_c3] -> Mux/3
  [v_c1] -> Mux1/1
  [w_c9] -> Mux/9
  [P_c8] -> Mux2/8
  [w_c1] -> Mux/1
  [w_c8] -> Mux/8
  [Vt4] -> Mux1/11
  [P_c9] -> Mux2/9
  [v_c6] -> Mux1/6
  [P_c1] -> Mux2/1
  [Vt1] -> Mux1/10
  [P_c6] -> Mux2/6
  [P_sm1] -> Mux2/10
  [P_c3] -> Mux2/3
  [P_c2] -> Mux2/2
  [w_sm1] -> Mux/10
  Mux/1 -> w/1
  Mux1/1 -> V/1
  Mux3/1 -> Terminator/1
  [w_c3] -> Mux4/3
  [w_sm1] -> Mux4/10
  [w_c5] -> Mux4/5
  [w_c2] -> Mux4/2
  [w_sm2] -> Mux4/11
  Mux4/1 -> Discrete Derivative/1
  [w_c8] -> Mux4/8
  [w_c6] -> Mux4/6
  [w_c9] -> Mux4/9
  [w_c7] -> Mux4/7
  [w_c4] -> Mux4/4
  [w_c1] -> Mux4/1
  Discrete Derivative/1 -> First-Order Filter/1
  First-Order Filter/1 -> dw/1

== system simulation_model_dynamic/Area 1/INVERTER 1 ==
  GFL1 : Subsystem  mask{Pnom=Sb, Vnom=Vb(1), Fnom=fb, Vdc_nom=Vdc(1), RLC_Filter=[r_f(1) l_f(1) c_f(1)], Pref=pset(1), Qref=qset(1), PLL_p=kp_pll(1), PLL_i=ki_pll(1), D_gfl=d_gfl(1), Voltage_P=kp_q(1), Voltage_I=ki_q(1), Current_P=kp_i(1), Current_I=ki_i(1), Power_P=kp_p(1), Power_I=ki_p(1), kf=1, InitialV=Init_GFL(1)}
      mask prompts: Pnom "Rated Power(VA)"; Vnom "Rated L-L RMS Voltage(V)"; Fnom "Rated Frequency(Hz)"; Vdc_nom "DC capacitor voltage(V)"; RLC_Filter "Grid-side coupling impedance(p.u.)"; Pref "Active Power Setting"; Qref "Reactive Power Setting"; PLL_p "PL Proportional Gain"; PLL_i "PLL Integral Gain"; D_gfl "Damping"; Voltage_P "Voltage Proportional Gain"; Voltage_I "Voltage Integral Gain"; Current_P "Current Proportional Gain"; Current_I "Current Integral Gain"; Power_P "Power Proportional Gain"; Power_I "Power Integral Gain"; kf "Feedforward Gain"; InitialV "Initial Condition"
      mask init:
      | R_f=RLC_Filter(1);
      | L_f=RLC_Filter(2);
      | C_f=RLC_Filter(3);
      mask Display: disp('GFL');
  Terminator : Terminator
  Terminator1 : Terminator
  A : PMIOPort  Side=Left
  B : PMIOPort  Port=2  Side=Left
  C : PMIOPort  Port=3  Side=Left
  tag scope: P_c1=global, Q_c1=global, v_c1=global, w_c1=global
  wires:
  GFL1/1(P) -> [P_c1]
  GFL1/2(Omega) -> [w_c1]
  GFL1/3(Vabs) -> [v_c1]
  GFL1/4(theta_t) -> Terminator/1
  GFL1/5(Q) -> [Q_c1]
  GFL1/6(theta_0) -> Terminator1/1
  connections:
  GFL1/RConn3 -- C/RConn1
  GFL1/RConn2 -- B/RConn1
  GFL1/RConn1 -- A/RConn1

== system simulation_model_dynamic/Area 1/INVERTER 2 ==
  GFM2 : Subsystem  mask{Sbnorm=Sb, Vbnorm=Vb_gfm, fbnorm=fb, Vdcnorm=Vdc_gfm(2), RLCnorm=[r_f_gfm(2) l_f_gfm(2) c_f_gfm(2)], P_setnorm=P_set_gfm(2), Q_setnorm=Q_set_gfm(2), Jnorm=J_gfm(2), Dpnorm=D_p_gfm(2), Dqnorm=D_q_gfm(2), Voltage_P=kp_vc_gfm(2), Voltage_I=ki_vc_gfm(2), Current_P=kp_i_gfm(2), Current_I=ki_i_gfm(2), InitialV=Init(2)}
      mask prompts: Sbnorm "Rated Power (VA)"; Vbnorm "Rated L-L RMS Voltage (V)"; fbnorm "Rated frequency (Hz)"; Vdcnorm "DC Voltage (V)"; RLCnorm "Grid-side coupling impedance (real)"; P_setnorm "Power Setting (W)"; Q_setnorm "Reactive Power Setting (W)"; Jnorm "Inertia"; Dpnorm "Power Damping"; Dqnorm "Reactive Power Droop"; Voltage_P "Voltage Proportional Gain"; Voltage_I "Voltage Integral Gain"; Current_P "Current Proportional Gain"; Current_I "Current Integral Gain"; InitialV "Initial Condition"
      mask Display: disp('GFM');
  Terminator : Terminator
  Terminator1 : Terminator
  fake_VSC : spsThreePhaseSourceLib/Three-Phase Source  Commented=on  InternalConnection=Yg  VoltagePhases=off  Voltage=(20000)*1  PhaseAngle=0  Voltage_phases=[25e3 25e3 25e3]/sqrt(3)  PhaseAngles_phases=[0 -120 +120]  Frequency=60  NonIdealSource=off  SpecifyImpedance=off  Resistance=0  Inductance=0  ShortCircuitLevel=100e6  BaseVoltage=20e3  XRratio=7  BusType=swing  Pref=1.0062*900e6  Qref=0  Prefabc=[10e3, 10e3, 10e3]  Qrefabc=[0, 0, 0]  Qmin=-inf  Qmax=inf
  A : PMIOPort  Side=Left
  B : PMIOPort  Port=2  Side=Left
  C : PMIOPort  Port=3  Side=Left
  tag scope: P_c2=global, Q_c2=global, v_c2=global, w_c2=global
  wires:
  GFM2/1(P) -> [P_c2]
  GFM2/3(Vabs) -> [v_c2]
  GFM2/5(theta_0) -> Terminator1/1
  GFM2/2(Omega) -> [w_c2]
  GFM2/4(theta_t) -> Terminator/1
  GFM2/6(Q) -> [Q_c2]
  connections:
  GFM2/RConn2 -- fake_VSC/RConn2 -- B/RConn1
  A/RConn1 -- fake_VSC/RConn1 -- GFM2/RConn1
  C/RConn1 -- fake_VSC/RConn3 -- GFM2/RConn3

== system simulation_model_dynamic/Area 1/INVERTER 3 ==
  GFM3 : Subsystem  mask{Sbnorm=Sb, Vbnorm=Vb_gfm, fbnorm=fb, Vdcnorm=Vdc_gfm(3), RLCnorm=[r_f_gfm(3) l_f_gfm(3) c_f_gfm(3)], P_setnorm=P_set_gfm(3), Q_setnorm=Q_set_gfm(3), Jnorm=J_gfm(3), Dpnorm=D_p_gfm(3), Dqnorm=D_q_gfm(3), Voltage_P=kp_vc_gfm(3), Voltage_I=ki_vc_gfm(3), Current_P=kp_i_gfm(3), Current_I=ki_i_gfm(3), InitialV=Init(3)}
      mask prompts: Sbnorm "Rated Power (VA)"; Vbnorm "Rated L-L RMS Voltage (V)"; fbnorm "Rated frequency (Hz)"; Vdcnorm "DC Voltage (V)"; RLCnorm "Grid-side coupling impedance (real)"; P_setnorm "Power Setting (W)"; Q_setnorm "Reactive Power Setting (W)"; Jnorm "Inertia"; Dpnorm "Power Damping"; Dqnorm "Reactive Power Droop"; Voltage_P "Voltage Proportional Gain"; Voltage_I "Voltage Integral Gain"; Current_P "Current Proportional Gain"; Current_I "Current Integral Gain"; InitialV "Initial Condition"
      mask Display: disp('GFM');
  Terminator : Terminator
  Terminator1 : Terminator
  fake_VSC : spsThreePhaseSourceLib/Three-Phase Source  Commented=on  InternalConnection=Yg  VoltagePhases=off  Voltage=(20000)*1  PhaseAngle=-12.1661  Voltage_phases=[25e3 25e3 25e3]/sqrt(3)  PhaseAngles_phases=[0 -120 +120]  Frequency=60  NonIdealSource=off  SpecifyImpedance=off  Resistance=0  Inductance=0  ShortCircuitLevel=100e6  BaseVoltage=20e3  XRratio=7  BusType=PV  Pref=200e6  Qref=0  Prefabc=[10e3, 10e3, 10e3]  Qrefabc=[0, 0, 0]  Qmin=-inf  Qmax=inf
  A : PMIOPort  Side=Left
  B : PMIOPort  Port=2  Side=Left
  C : PMIOPort  Port=3  Side=Left
  tag scope: P_c3=global, Q_c3=global, v_c3=global, w_c3=global
  wires:
  GFM3/5(theta_0) -> Terminator1/1
  GFM3/2(Omega) -> [w_c3]
  GFM3/4(theta_t) -> Terminator/1
  GFM3/6(Q) -> [Q_c3]
  GFM3/3(Vabs) -> [v_c3]
  GFM3/1(P) -> [P_c3]
  connections:
  C/RConn1 -- fake_VSC/RConn3 -- GFM3/RConn3
  B/RConn1 -- fake_VSC/RConn2 -- GFM3/RConn2
  A/RConn1 -- fake_VSC/RConn1 -- GFM3/RConn1

== system simulation_model_dynamic/Area 1/M1: Turbine & Regulators ==
  note: MACHINE 1
  m : Inport
  Pref : Inport  Port=2
  Vref : Inport  Port=3
  PSS : Inport  Port=4
  Bus Selector : BusSelector  OutputSignals="dq0 components.Stator voltage  vd (pu),dq0 components.Stator voltage  vq (pu),Mechanical.Rotor angle deviation  d_theta (rad),Mechanical.Rotor speed  wm  (pu),Mechanical.Electrical power  Pe (pu),Mechanical.Rotor speed deviation  dw (pu),Mechanical.Rotor mechanical angle  theta (deg)"
  Complex to Magnitude-Angle : ComplexToMagnitudeAngle  Output=Magnitude
  "Delta Pa PSS " : spsGenericPowerSystemStabilizerLib/Generic Power System Stabilizer  Tsensor=15e-3  K=2.5*1.25  Twashout=1  Tleadlag1=[60e-3 1]  Tleadlag2=[0 0]  VSlimits=[-0.15 0.15]  Vinit=0  Plot_On=off  MagdB_On=off  FreqRange=logspace(-2,2,500)
      settings: LibrarySourceBlock=|
      | sps_lib/Electrical Machines/Synchronous Machine Control/Generic
      | Power System Stabilizer
  "Delta w PSS (Kundur) " : spsGenericPowerSystemStabilizerLib/Generic Power System Stabilizer  Tsensor=15e-3  K=30  Twashout=10  Tleadlag1=[50e-3 20e-3]  Tleadlag2=[3 5.4]  VSlimits=[-0.15 0.15]  Vinit=0  Plot_On=off  MagdB_On=off  FreqRange=logspace(-2,2,500)
      settings: LibrarySourceBlock=|
      | sps_lib/Electrical Machines/Synchronous Machine Control/Generic
      | Power System Stabilizer
  EXCITATION : spsExcitationSystemLib/Excitation System  tr=20e-3  reg=[ 200, 0.001 ]  exc=[ 1, 0 ]  tgr=[ 0, 0 ]  damp=[ 0, 0 ]  sat=[ 0, 0 ]  lim=[ 0 , 12.3, 0 ]  v0=[1 1.4305]
      settings: LibrarySourceBlock=sps_lib/Electrical Machines/Synchronous Machine Control/Excitation System
  "MB-PSS " : spsMultiBandPowerSystemStabilizerLib/Multi-Band Power System Stabilizer  OperationMode=Simplified settings  Kg=1.0  GL=[0.2 30]  GI=[1.25 40]  GH=[12.0 160]  GLd=[66 66 9.4]  TcLF=[1.667 2 0 0 0 0 2 2.4 0 0 0 0 1 1]  GId=[66 66 47.6]  TcIF=[1 1 0.25 0.3 0 0 1 1 0.3 0.36 0 0 0 0]  GHd=[66 66 233]  TcHF="[0.01 0.012 0 0 0 0  0.012 0.0144 0 0 0 0 1 1]"  LIM=[.075 .15 .15 .15]  Plot_On=off  MagdB_On=off  FreqRange=logspace(-2,2,500)
      settings: LibrarySourceBlock=|
      | sps_lib/Electrical Machines/Synchronous Machine Control/Multi-Band
      | Power System Stabilizer
  Multiport Switch : MultiPortSwitch  Inputs=4  SaturateOnIntegerOverflow=off
  PSS model1 : Constant  Value=0
  PSS model2 : Constant
  Real-Imag to Complex : RealImagToComplex
  STG : spsSteamTurbineandGovernorLib/Steam Turbine and Governor  gentype=Tandem-compound (single mass)  reg1="[ 1 10    0 ]"  reg2="[ 0.001  0.15 ]"  reg3="[ -0.1  0.1  0  4.496 ]"  N=3600  turb1="[ 0  10   3.3   0.5   ]"  turb2="[   0   0.36    0.36   0.28   ]"  HA="[ 0.046  1.430  1.465   0.192 ]"  KA="[ 90.44  53.88  64.59   62.94  ]"  DA="[ 0.0115  0.3575  0.3663   0.0137  ]"  ini1=0.50063  ini2=[0.779316,-31.4247]
      settings: LibrarySourceBlock=|
      | sps_lib/Electrical Machines/Synchronous Machine Control/Steam Turbine
      | and Governor
  Sum1 : Sum  InputSameDT=on  SaturateOnIntegerOverflow=on  OutDataTypeStr=Inherit: Same as first input
  Sum2 : Sum  Inputs=-+  InputSameDT=on  SaturateOnIntegerOverflow=on  OutDataTypeStr=Inherit: Same as first input
  Terminator : Terminator
  Terminator1 : Terminator
  Terminator2 : Terminator
  wref : Constant
  Pm : Outport  InitialOutput=0  VectorParamsAs1DForOutWhenUnconnected=off
  Vf : Outport  Port=2  InitialOutput=0  VectorParamsAs1DForOutWhenUnconnected=off
  tag scope: EFD1=global, Pa1=global, Pe1=global, Vt1=global, pss1=global, theta1=global, w1=global
  wires:
  Bus Selector/1 -> Real-Imag to Complex/1, EXCITATION/2  "<Stator voltage  vd (pu)>"
  Bus Selector/2 -> Real-Imag to Complex/2, EXCITATION/3  "<Stator voltage  vq (pu)>"
  wref/1 -> STG/1
  Pref/1 -> STG/2
  m/1 -> Bus Selector/1
  Vref/1 -> EXCITATION/1
  Real-Imag to Complex/1 -> Complex to Magnitude-Angle/1
  EXCITATION/1 -> Vf/1, [EFD1]
  Complex to Magnitude-Angle/1 -> [Vt1]
  Bus Selector/7 -> [theta1]  "<Rotor mechanical angle  theta (deg)>"
  Multiport Switch/1 -> EXCITATION/4, [pss1]
  PSS model1/1 -> Multiport Switch/2
  "MB-PSS "/1 -> Multiport Switch/3
  "Delta w PSS (Kundur) "/1 -> Multiport Switch/4
  "Delta Pa PSS "/1 -> Multiport Switch/5
  PSS model2/1 -> Sum1/2
  Sum1/1 -> Multiport Switch/1
  PSS/1 -> Sum1/1
  Bus Selector/4 -> [w1], STG/3  "<Rotor speed  wm  (pu)>"
  Bus Selector/5 -> [Pe1], Sum2/1  "<Electrical power  Pe (pu)>"
  Bus Selector/6 -> "Delta w PSS (Kundur) "/1, "MB-PSS "/1  "<Rotor speed deviation  dw (pu)>"
  Sum2/1 -> [Pa1], "Delta Pa PSS "/1  "Pm-Pe"
  STG/3 -> Terminator/1
  STG/4 -> Pm/1, Sum2/2
  STG/2 -> Terminator1/1
  STG/1 -> Terminator2/1
  Bus Selector/3 -> STG/4  "<Rotor angle deviation  d_theta (rad)>"

== system simulation_model_dynamic/Area 2/INVERTER 4 ==
  GFM4 : Subsystem  mask{Sbnorm=Sb, Vbnorm=Vb_gfm, fbnorm=fb, Vdcnorm=Vdc_gfm(4), RLCnorm=[r_f_gfm(4) l_f_gfm(4) c_f_gfm(4)], P_setnorm=P_set_gfm(4), Q_setnorm=Q_set_gfm(4), Jnorm=J_gfm(4), Dpnorm=D_p_gfm(4), Dqnorm=D_q_gfm(4), Voltage_P=kp_vc_gfm(4), Voltage_I=ki_vc_gfm(4), Current_P=kp_i_gfm(4), Current_I=ki_i_gfm(4), InitialV=Init(4)}
      mask prompts: Sbnorm "Rated Power (VA)"; Vbnorm "Rated L-L RMS Voltage (V)"; fbnorm "Rated frequency (Hz)"; Vdcnorm "DC Voltage (V)"; RLCnorm "Grid-side coupling impedance (real)"; P_setnorm "Power Setting (W)"; Q_setnorm "Reactive Power Setting (W)"; Jnorm "Inertia"; Dpnorm "Power Damping"; Dqnorm "Reactive Power Droop"; Voltage_P "Voltage Proportional Gain"; Voltage_I "Voltage Integral Gain"; Current_P "Current Proportional Gain"; Current_I "Current Integral Gain"; InitialV "Initial Condition"
      mask Display: disp('GFM');
  Terminator : Terminator
  Terminator1 : Terminator
  fake_VSC : spsThreePhaseSourceLib/Three-Phase Source  Commented=on  InternalConnection=Yg  VoltagePhases=off  Voltage=(20000)*1  PhaseAngle=-21.2528  Voltage_phases=[25e3 25e3 25e3]/sqrt(3)  PhaseAngles_phases=[0 -120 +120]  Frequency=60  NonIdealSource=off  SpecifyImpedance=off  Resistance=0  Inductance=0  ShortCircuitLevel=100e6  BaseVoltage=20e3  XRratio=7  BusType=PV  Pref=550e6  Qref=0  Prefabc=[10e3, 10e3, 10e3]  Qrefabc=[0, 0, 0]  Qmin=-inf  Qmax=inf
  A : PMIOPort  Side=Left
  B : PMIOPort  Port=2  Side=Left
  C : PMIOPort  Port=3  Side=Left
  tag scope: P_c4=global, Q_c4=global, v_c4=global, w_c4=global
  wires:
  GFM4/6(Q) -> [Q_c4]
  GFM4/4(theta_t) -> Terminator/1
  GFM4/2(Omega) -> [w_c4]
  GFM4/5(theta_0) -> Terminator1/1
  GFM4/1(P) -> [P_c4]
  GFM4/3(Vabs) -> [v_c4]
  connections:
  GFM4/RConn2 -- fake_VSC/RConn2 -- B/RConn1
  GFM4/RConn1 -- fake_VSC/RConn1 -- A/RConn1
  C/RConn1 -- fake_VSC/RConn3 -- GFM4/RConn3
